simulink model "first_order_process-MESSEDUP"  (R2013a)
settings: Solver=ode3  StartTime=0  StopTime=1  RelTol=1e-3
values from neighbouring files (symbols this model uses):
  SAMPLING_INTERVAL = 10    [main_code.m]    (also in main_using_Torsche.m)
  StartTime = task{subtask_num}.start_time    [main_code.m]    (also in main_using_Torsche.m = task(subtask_num).start_time)
  x_initial_product_setpoint = last_setpoint    [main_code.m]    (also in main_using_Torsche.m)
  x_new_product_setpoint = task{subtask_num}.set_point    [main_code.m]    (also in main_using_Torsche.m = task(subtask_num).set_point)
  x_product_id = task{subtask_num}.product_id    [main_code.m]    (also in main_using_Torsche.m = task(subtask_num).product_id)
  x_throughput_setpoint = task{subtask_num}.speed    [main_code.m]    (also in main_using_Torsche.m = task(subtask_num).speed)
libraries: simulink x1
settings Model: Creator=acer  LastModifiedBy=acer
settings OptimizationCC: SimCompilerOptimization=On
settings HardwareCC: ProdBitPerInt=16  ProdBitPerPointer=8  ProdIntDivRoundTo=Zero  ProdWordSize=8  ProdShiftRightIntArith=off  ProdHWDeviceType=Intel->8051 Compatible
settings RTWCC: RTWCompilerOptimization=On

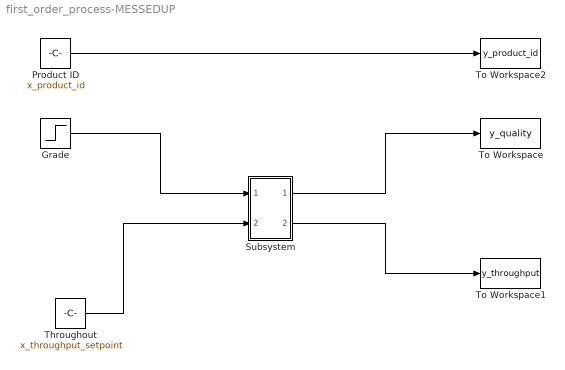
== system first_order_process-MESSEDUP ==
  Grade : Step  Time=StartTime + SAMPLING_INTERVAL  Before=x_initial_product_setpoint  After=x_new_product_setpoint  SampleTime=0
  Product ID : Constant  Value=x_product_id
  Subsystem : Subsystem
  Throughout : Constant  Value=x_throughput_setpoint
  To Workspace : ToWorkspace  VariableName=y_quality  SampleTime=SAMPLING_INTERVAL  SaveFormat=Timeseries
  To Workspace1 : ToWorkspace  VariableName=y_throughput  SampleTime=SAMPLING_INTERVAL  SaveFormat=Timeseries
  To Workspace2 : ToWorkspace  VariableName=y_product_id  SampleTime=SAMPLING_INTERVAL  SaveFormat=Timeseries
  wires:
  Product ID/1 -> To Workspace2/1
  Grade/1 -> Subsystem/1(In1)
  Throughout/1 -> Subsystem/2(In2)
  Subsystem/1(Out1) -> To Workspace/1
  Subsystem/2(Out2) -> To Workspace1/1

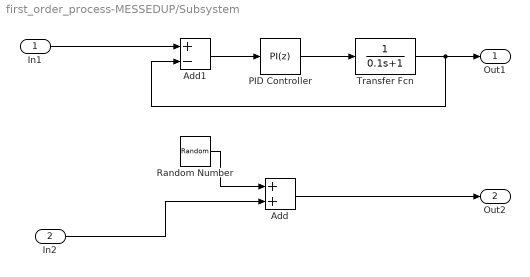
== system first_order_process-MESSEDUP/Subsystem ==
  In1 : Inport
  In2 : Inport  Port=2
  Add : Sum  SampleTime=SAMPLING_INTERVAL
  Add1 : Sum  Inputs=+-  SampleTime=SAMPLING_INTERVAL
  PID Controller : simulink/Continuous/PID Controller  Controller=PI  TimeDomain=Discrete-time  SampleTime=SAMPLING_INTERVAL  IntegratorMethod=Forward Euler  FilterMethod=Forward Euler  Form=Ideal  P=.01  I=40  D=0  N=100  InitialConditionSource=internal  InitialConditionForIntegrator=0  InitialConditionForFilter=0  ExternalReset=none  LimitOutput=off  UpperSaturationLimit=inf  LowerSaturationLimit=-inf  LinearizeAsGain=on  AntiWindupMode=none  Kb=1  TrackingMode=off  Kt=1  PParamMin=[]  PParamMax=[]  IParamMin=[]  IParamMax=[]  DParamMin=[]  DParamMax=[]  NParamMin=[]  NParamMax=[]  KbParamMin=[]  KbParamMax=[]  KtParamMin=[]  KtParamMax=[]  POutMin=[]  POutMax=[]  IOutMin=[]  IOutMax=[]  DOutMin=[]  DOutMax=[]  NOutMin=[]  NOutMax=[]  KbOutMin=[]  KbOutMax=[]  KtOutMin=[]  KtOutMax=[]  IntegratorOutMin=[]  IntegratorOutMax=[]  FilterOutMin=[]  FilterOutMax=[]  SumOutMin=[]  SumOutMax=[]  SumI1OutMin=[]  SumI1OutMax=[]  SumI2OutMin=[]  SumI2OutMax=[]  SumI3OutMin=[]  SumI3OutMax=[]  SumDOutMin=[]  SumDOutMax=[]  SaturationOutMin=[]  SaturationOutMax=[]  IntegratorContinuousStateAttributes=''  IntegratorStateMustResolveToSignalObject=off  IntegratorRTWStateStorageClass=Auto  FilterContinuousStateAttributes=''  FilterStateMustResolveToSignalObject=off  FilterRTWStateStorageClass=Auto
  Random Number : RandomNumber  SampleTime=SAMPLING_INTERVAL
  Transfer Fcn : TransferFcn  Denominator=[0.1 1]
  Out1 : Outport
  Out2 : Outport  Port=2
  wires:
  Transfer Fcn/1 -> Add1/2, Out1/1
  Random Number/1 -> Add/1
  In2/1 -> Add/2
  Add/1 -> Out2/1
  PID Controller/1 -> Transfer Fcn/1
  In1/1 -> Add1/1
  Add1/1 -> PID Controller/1
